simulink model "TP1105Son"  (R2019a)
settings: Solver=VariableStepAuto  StartTime=0.0  StopTime=3  RelTol=1e-3
libraries: dspobslib x2, dspvision x1
settings Model: Creator=28610075  LastModifiedBy=28610075

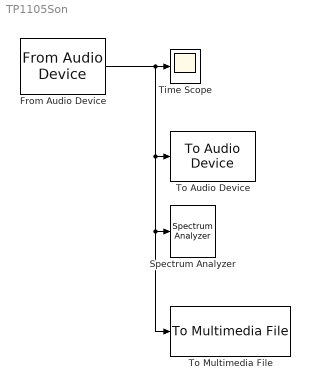
== system TP1105Son ==
  From Audio Device : dspobslib/From Audio Device  deviceName=Default  numChannels=1  sampleRate=80000  deviceDatatype=Determine from output data type  autoBufferSize=on  bufferSize=4096  queueDuration=1.0  frameSize=1024  outputDatatype=double  defaultInputChannelMapping=on  inputChannelMapping=1:2  outputNumOverrunSamples=off  OutputFrames=on
      settings: SourceProductName=DSP System Toolbox  SourceProductBaseCode=DS
  Spectrum Analyzer : SpectrumAnalyzer
  Time Scope : Scope
  To Audio Device : dspobslib/To Audio Device  deviceName=Default  inheritSampleRate=on  sampleRate=44100  deviceDatatype=Determine from input data type  autoBufferSize=on  bufferSize=4096  queueDuration=5  defaultOutputChannelMapping=on  outputChannelMapping=1:2  outputNumUnderrunSamples=off
      settings: SourceProductName=DSP System Toolbox  SourceProductBaseCode=DS
  To Multimedia File : dspvision/To Multimedia File  outputFilename=lect4.wav  streamSelection=Audio only  videoCompressor=None (uncompressed)  audioCompressor=None (uncompressed)  imagePorts=Separate color signals  fileType=WAV  audioDatatype=16-bit integer  fourcc=RGB  videoQuality=75  mj2000CompFactor=10
      settings: SourceProductName=DSP System Toolbox  SourceProductBaseCode=DS
  wires:
  From Audio Device/1 -> To Multimedia File/1, Spectrum Analyzer/1, To Audio Device/1, Time Scope/1
